simulink model "Go_Kart_Model"  (R2020b)
settings: Solver=VariableStepAuto  StartTime=0.0  StopTime=10  RelTol=1e-3
model workspace (MAT data in the model file):
  Air_Resistance = Simulink.Parameter
  Air_Resistance.Value = 0.26903
  Air_Resistance.DataType = 'auto'
  Air_Resistance.Dimensions = [1 1]
  Gear_Ratio = Simulink.Parameter
  Gear_Ratio.Value = 12.75
  Gear_Ratio.DataType = 'auto'
  Gear_Ratio.Dimensions = [1 1]
  Mass = Simulink.Parameter
  Mass.Value = 200
  Mass.DataType = 'auto'
  Mass.Dimensions = [1 1]
  Num_Motors = Simulink.Parameter
  Num_Motors.Value = 6
  Num_Motors.DataType = 'auto'
  Num_Motors.Dimensions = [1 1]
  Tire_Radius = Simulink.Parameter
  Tire_Radius.Value = 0.2286
  Tire_Radius.DataType = 'auto'
  Tire_Radius.Dimensions = [1 1]
settings Model: OrderedModelArguments=off  Creator=hanso  LastModifiedBy=hanso
settings DataIOCC: ReturnWorkspaceOutputs=off
settings DebuggingCC: ArithmeticOperatorsInVariantConditions=warning
settings SFSimCC: CustomCodeUndefinedFunction=UseInterfaceOnly

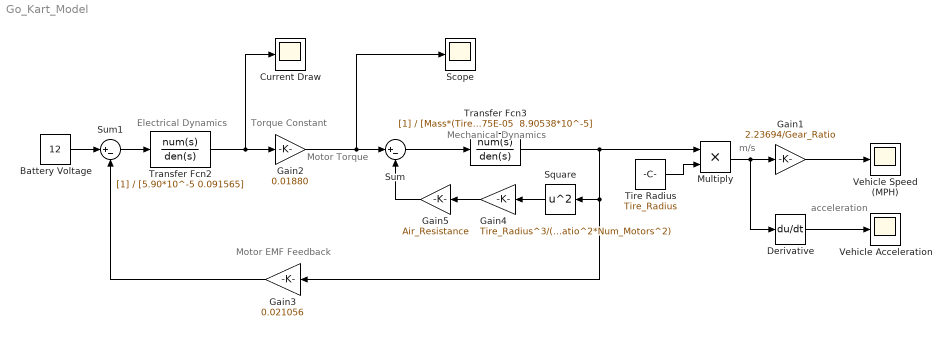
== system Go_Kart_Model ==
  note: acceleration
  note: m/s
  note: Torque Constant
  note: Electrical Dynamics
  note: Mechanical Dynamics
  note: Motor Torque
  note: Motor EMF Feedback
  Battery Voltage : Constant  Value=12
  Current Draw : Scope
  Derivative : Derivative
  Gain1 : Gain  Gain=2.23694/Gear_Ratio
  Gain2 : Gain  Gain=0.01880
  Gain3 : Gain  Gain=0.021056
  Gain4 : Gain  Gain=Tire_Radius^3/(Gear_Ratio^2*Num_Motors^2)
  Gain5 : Gain  Gain=Air_Resistance
  Multiply : Product
  Scope : Scope
  Square : Math  Operator=square  SignedPower=on  SaturateOnIntegerOverflow=on
  Sum : Sum  Inputs=|+-
  Sum1 : Sum  Inputs=|+-
  Tire Radius : Constant  Value=Tire_Radius
  Transfer Fcn2 : TransferFcn  Denominator=[5.90*10^-5 0.091565]
  Transfer Fcn3 : TransferFcn  Denominator=|
      | [Mass*(Tire_Radius)^2/(Gear_Ratio^2*Num_Motors^2)+7.75E-05
      | 
      |  8.90538*10^-5]
  Vehicle Acceleration : Scope
  Vehicle Speed (MPH) : Scope
  wires:
  Gain3/1 -> Sum1/2
  Sum1/1 -> Transfer Fcn2/1
  Tire Radius/1 -> Multiply/2
  Multiply/1 -> Derivative/1, Gain1/1
  Gain1/1 -> Vehicle Speed (MPH)/1
  Battery Voltage/1 -> Sum1/1
  Derivative/1 -> Vehicle Acceleration/1
  Transfer Fcn2/1 -> Current Draw/1, Gain2/1
  Sum/1 -> Transfer Fcn3/1
  Transfer Fcn3/1 -> Gain3/1, Square/1, Multiply/1
  Square/1 -> Gain4/1
  Gain5/1 -> Sum/2
  Gain4/1 -> Gain5/1
  Gain2/1 -> Scope/1, Sum/1
